simulink model "filter_IIR"  (Simulink 7.9)
settings: Solver=ode3  StartTime=0.0  StopTime=20  FixedStep=0.125e-3  RelTol=1e-3
libraries: simulink x1
settings Model: Creator=asus  LastModifiedBy=asus

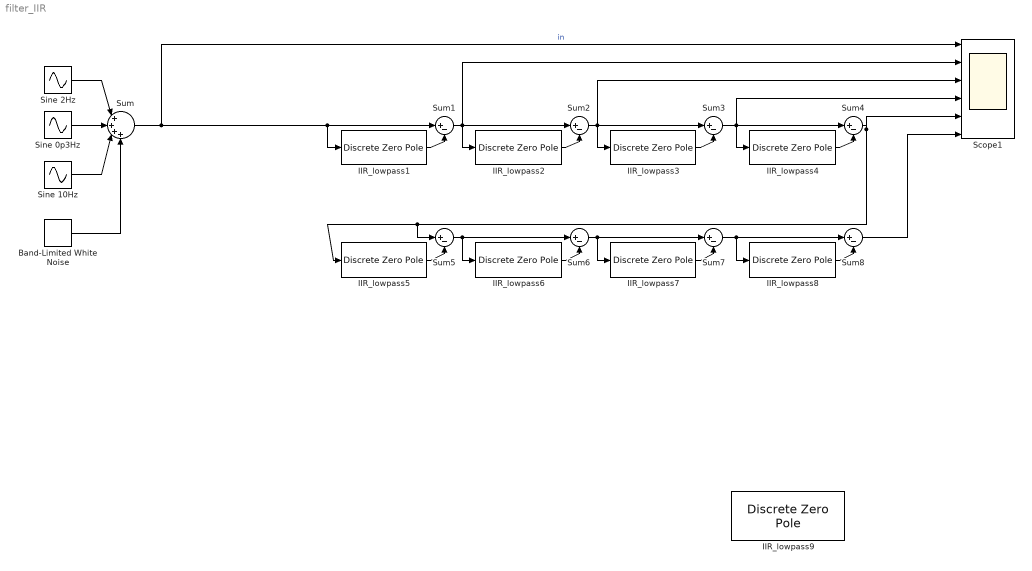
== system filter_IIR ==
  Band-Limited White Noise : simulink/Sources/Band-Limited White Noise  Cov=[1.25e-7]  Ts=0.125e-3  seed=[23341]
  IIR_lowpass{1..8} (8 alike) : DiscreteZeroPole  Zeros=[0]  Poles=4095/4096  Gain=1/4096  SampleTime=0.125e-3
  IIR_lowpass9 : DiscreteZeroPole  Zeros=zeros(1,5)  Poles=255/256*ones(1,5)  Gain=(1/256)^5*2^3  SampleTime=0.125e-3
  Scope1 : Scope  NumInputPorts=6
      settings: ShowLegends=on  TimeRange=20  YMin=-5~-2~-1~-5~-5~-5  YMax=5~2~1~5~5~5  MaxDataPoints=65536  SampleInput=on  SampleTime=0.125e-3
  Sine 0p3Hz : Sin  Amplitude=2  Frequency=0.3*2*pi  SampleTime=0.125e-3
  Sine 10Hz : Sin  Amplitude=0.1  Frequency=10*2*pi  SampleTime=0.125e-3
  Sine 2Hz : Sin  Amplitude=20e-3  Frequency=2*2*pi  SampleTime=0.125e-3
  Sum : Sum  Inputs=|++++  SampleTime=0.125e-3
  Sum{1..8} (8 alike) : Sum  Inputs=|+-
  wires:
  Sum/1 -> Scope1/1, IIR_lowpass1/1, Sum1/1  "in"
  IIR_lowpass1/1 -> Sum1/2
  Sum1/1 -> IIR_lowpass2/1, Sum2/1, Scope1/2
  Sine 2Hz/1 -> Sum/1
  Sine 0p3Hz/1 -> Sum/2
  Sine 10Hz/1 -> Sum/3
  Band-Limited White Noise/1 -> Sum/4
  IIR_lowpass2/1 -> Sum2/2
  Sum2/1 -> IIR_lowpass3/1, Sum3/1, Scope1/3
  IIR_lowpass3/1 -> Sum3/2
  Sum3/1 -> IIR_lowpass4/1, Sum4/1, Scope1/4
  IIR_lowpass4/1 -> Sum4/2
  IIR_lowpass5/1 -> Sum5/2
  Sum5/1 -> IIR_lowpass6/1, Sum6/1
  IIR_lowpass6/1 -> Sum6/2
  Sum6/1 -> IIR_lowpass7/1, Sum7/1
  IIR_lowpass7/1 -> Sum7/2
  Sum7/1 -> IIR_lowpass8/1, Sum8/1
  IIR_lowpass8/1 -> Sum8/2
  Sum4/1 -> IIR_lowpass5/1, Sum5/1, Scope1/5
  Sum8/1 -> Scope1/6
